simulink model "qcm_passband"  (R2026a)
settings: Solver=VariableStepAuto  StopTime=1
model workspace (MAT data in the model file):
  FrameSize = 1000
  Fs = 100000
libraries: dspsrcs4 x4, dspfdesign x2, commchan3 x1
settings Model: Creator=ranja  LastModifiedBy=ranja

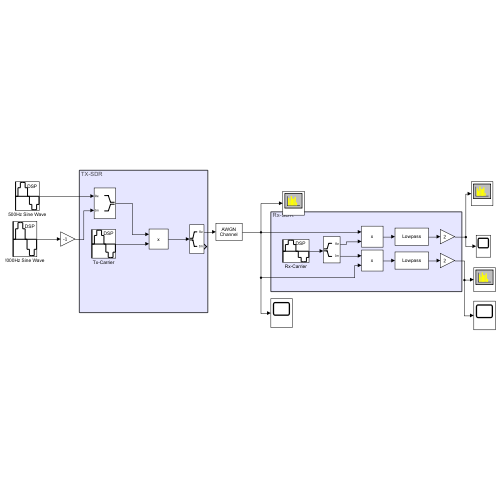
[thumbnail: Simulink's stored preview of the top-level diagram]
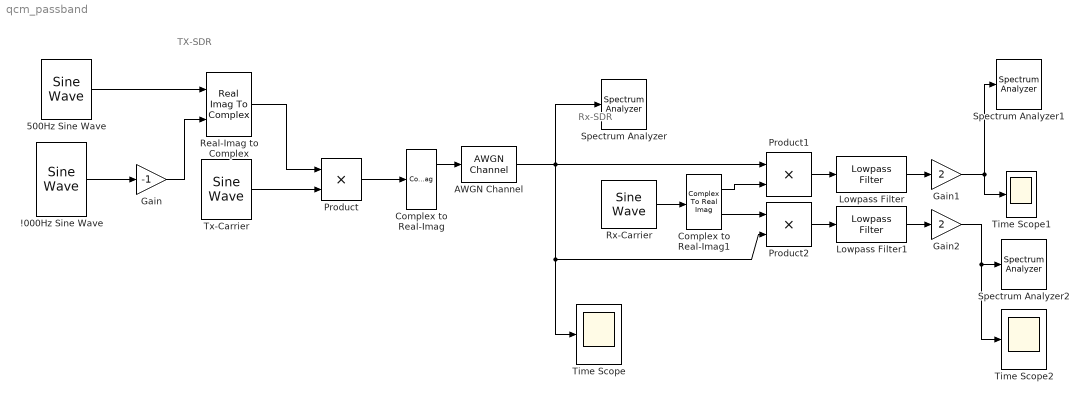
== system qcm_passband ==
  note: TX-SDR
  note: Rx-SDR
  !000Hz Sine Wave : dspsrcs4/Sine Wave  Amplitude=1  Frequency=1000  Phase=0  SampleMode=Discrete  OutComplex=Real  CompMethod=Trigonometric fcn  TableSize=Speed  SampleTime=1/Fs  SamplesPerFrame=FrameSize  ResetState=Restart at time zero  OutputFrames=off  dataType=double  wordLen=16  udDataType=sfix(16)  fracBitsMode=Best precision  numFracBits=15  OutDataTypeStr=double  LastOutDataTypeStr=double
  500Hz Sine Wave : dspsrcs4/Sine Wave  Amplitude=1  Frequency=500  Phase=0  SampleMode=Discrete  OutComplex=Real  CompMethod=Trigonometric fcn  TableSize=Speed  SampleTime=1/Fs  SamplesPerFrame=FrameSize  ResetState=Restart at time zero  OutputFrames=off  dataType=double  wordLen=16  udDataType=sfix(16)  fracBitsMode=Best precision  numFracBits=15  OutDataTypeStr=double  LastOutDataTypeStr=double
  AWGN Channel : commchan3/AWGN Channel  LegacyMode=off  NoiseMethod="Signal to noise ratio  (SNR)"  noiseMode="Signal to noise ratio  (SNR)"  EbNo=10  EsNo=10  SNR=20  BitsPerSymbol=1  SignalPower=1  SpecifySymbolPeriod=off  SamplesPerSymbol=1  SymbolPeriod=1  VarianceSource=Parameter  Variance=1  RandomStream=Global stream  Seed=67  SimulateUsing=Code generation
  Complex to Real-Imag : ComplexToRealImag
  Complex to Real-Imag1 : ComplexToRealImag
  Gain : Gain  Gain=-1
  Gain1 : Gain  Gain=2
  Gain2 : Gain  Gain=2
  Lowpass Filter : dspfdesign/Lowpass Filter  FilterType=FIR  DesignForMinimumOrder=off  FilterOrder=50  PassbandFrequency=1500  StopbandFrequency=0.5442  PassbandRipple=0.1  StopbandAttenuation=80  SampleRateMode=Specify on dialog  SampleRate=Fs  SimulateUsing=Interpreted execution  roundingMode=Floor  coeffsDataTypeStr=fixdt(1,16)
  Lowpass Filter1 : dspfdesign/Lowpass Filter  FilterType=FIR  DesignForMinimumOrder=off  FilterOrder=50  PassbandFrequency=1500  StopbandFrequency=0.5442  PassbandRipple=0.1  StopbandAttenuation=80  SampleRateMode=Specify on dialog  SampleRate=Fs  SimulateUsing=Interpreted execution  roundingMode=Floor  coeffsDataTypeStr=fixdt(1,16)
  Product : Product
  Product1 : Product
  Product2 : Product  Inputs=2
  Real-Imag to Complex : RealImagToComplex
  Rx-Carrier : dspsrcs4/Sine Wave  Amplitude=1  Frequency=10000+50  Phase=pi/6  SampleMode=Discrete  OutComplex=Complex  CompMethod=Trigonometric fcn  TableSize=Speed  SampleTime=1/Fs  SamplesPerFrame=FrameSize  ResetState=Restart at time zero  OutputFrames=off  dataType=double  wordLen=16  udDataType=sfix(16)  fracBitsMode=Best precision  numFracBits=15  OutDataTypeStr=double  LastOutDataTypeStr=double
  Spectrum Analyzer : SpectrumAnalyzer  WindowInvariantSamplesPerUpdate=on
  Spectrum Analyzer1 : SpectrumAnalyzer  WindowInvariantSamplesPerUpdate=on
  Spectrum Analyzer2 : SpectrumAnalyzer  WindowInvariantSamplesPerUpdate=on
  Time Scope : Scope
      settings: TimeUnits=Metric (based on Time Span)  ActiveDisplayYMinimum=-1.9395106260328816  ActiveDisplayYMaximum=1.9155010383387165  YLabel=Amplitude
  Time Scope1 : Scope
      settings: TimeUnits=Metric (based on Time Span)  ActiveDisplayYMinimum=-1.5451049392652738  ActiveDisplayYMaximum=1.3180434959411933  YLabel=Amplitude
  Time Scope2 : Scope
      settings: TimeUnits=Metric (based on Time Span)  ActiveDisplayYMinimum=-1.692420845147262  ActiveDisplayYMaximum=1.6853688071586088  YLabel=Amplitude  DataLoggingVariableName=ScopeData2
  Tx-Carrier : dspsrcs4/Sine Wave  Amplitude=1  Frequency=10000  Phase=0  SampleMode=Discrete  OutComplex=Complex  CompMethod=Trigonometric fcn  TableSize=Speed  SampleTime=1/Fs  SamplesPerFrame=FrameSize  ResetState=Restart at time zero  OutputFrames=off  dataType=double  wordLen=16  udDataType=sfix(16)  fracBitsMode=Best precision  numFracBits=15  OutDataTypeStr=double  LastOutDataTypeStr=double
  wires:
  !000Hz Sine Wave/1 -> Gain/1
  500Hz Sine Wave/1 -> Real-Imag to Complex/1
  Gain/1 -> Real-Imag to Complex/2
  Real-Imag to Complex/1 -> Product/1
  Tx-Carrier/1 -> Product/2
  Product/1 -> Complex to Real-Imag/1
  Complex to Real-Imag1/2 -> Product2/1
  Rx-Carrier/1 -> Complex to Real-Imag1/1
  Complex to Real-Imag1/1 -> Product1/2
  Product1/1 -> Lowpass Filter/1
  Product2/1 -> Lowpass Filter1/1
  Lowpass Filter/1 -> Gain1/1
  Lowpass Filter1/1 -> Gain2/1
  Gain1/1 -> Spectrum Analyzer1/1, Time Scope1/1
  Gain2/1 -> Spectrum Analyzer2/1, Time Scope2/1
  Complex to Real-Imag/1 -> AWGN Channel/1
  AWGN Channel/1 -> Spectrum Analyzer/1, Time Scope/1, Product2/2, Product1/1
